simulink model "chap7_9sim"  (Simulink 5.0)
settings: Solver=ode45  StartTime=0.0  StopTime=6  RelTol=1e-3
settings Model: LastModifiedBy=Administrator

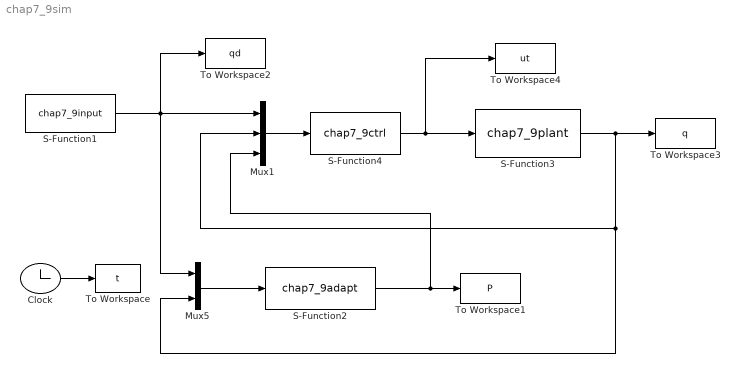
== system chap7_9sim ==
  Clock : Clock
      settings: Decimation=10
  Mux1 : Mux  Inputs=3
  Mux5 : Mux  Inputs=2
  S-Function1 : S-Function  FunctionName=chap7_9input
  S-Function2 : S-Function  FunctionName=chap7_9adapt
  S-Function3 : S-Function  FunctionName=chap7_9plant
  S-Function4 : S-Function  FunctionName=chap7_9ctrl
  To Workspace : ToWorkspace  VariableName=t  SampleTime=-1  SaveFormat=Array
  To Workspace1 : ToWorkspace  VariableName=P  SampleTime=-1  SaveFormat=Array
  To Workspace2 : ToWorkspace  VariableName=qd  SampleTime=-1  SaveFormat=Array
  To Workspace3 : ToWorkspace  VariableName=q  SampleTime=-1  SaveFormat=Array
  To Workspace4 : ToWorkspace  VariableName=ut  SampleTime=-1  SaveFormat=Array
  wires:
  S-Function4/1 -> S-Function3/1, To Workspace4/1
  S-Function3/1 -> Mux5/2, Mux1/2, To Workspace3/1
  Mux5/1 -> S-Function2/1
  Mux1/1 -> S-Function4/1
  S-Function1/1 -> Mux1/1, Mux5/1, To Workspace2/1
  S-Function2/1 -> To Workspace1/1, Mux1/3
  Clock/1 -> To Workspace/1
